simulink model "Sine_wave"  (R2022b)
settings: Solver=VariableStepAuto  StartTime=0.0  StopTime=10.0  RelTol=1e-3
libraries: simulink x1
settings Model: Creator=poorn  LastModifiedBy=poorn

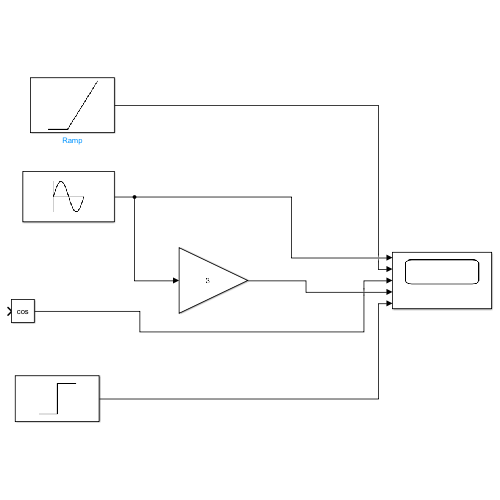
[thumbnail: Simulink's stored preview of the top-level diagram]
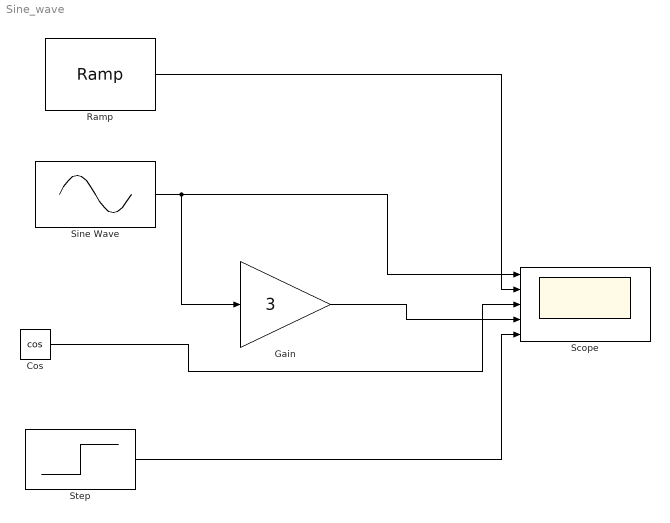
== system Sine_wave ==
  Cos : Trigonometry  Operator=cos
  Gain : Gain  Gain=3
  Ramp : simulink/Sources/Ramp  slope=1  start=0  InitialOutput=0
  Scope : Scope  NumInputPorts=5
  Sine Wave : Sin  SampleTime=0
  Step : Step  SampleTime=0
  wires:
  Sine Wave/1 -> Scope/1, Gain/1
  Gain/1 -> Scope/4
  Step/1 -> Scope/5
  Ramp/1 -> Scope/2
  Cos/1 -> Scope/3
